simulink model "Manipulator_AdaptiveInverseDynamics"  (R2022b)
settings: Solver=FixedStepAuto  StartTime=0.0  StopTime=t_final  FixedStep=dt  RelTol=1e-3
values from neighbouring files (symbols this model uses):
  dt = 1.00e-03    (= 0.001)    [Initialization.m]
  Kd = 50*eye(3,3)    [AdaptiveInverseDynamicsInit.m]
  Kp = 20*eye(3,3)    [AdaptiveInverseDynamicsInit.m]
  P = lyap(A', Q)    [AdaptiveInverseDynamicsInit.m]
  theta_params_init = [p1;p2;p3;p4;p5;p6]    [AdaptiveInverseDynamicsInit.m]
libraries: simulink x3
settings Model: Creator=lukasz  LastModifiedBy=lukasz

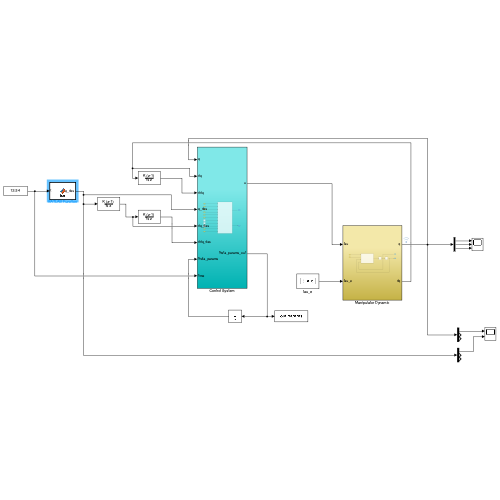
[thumbnail: Simulink's stored preview of the top-level diagram]
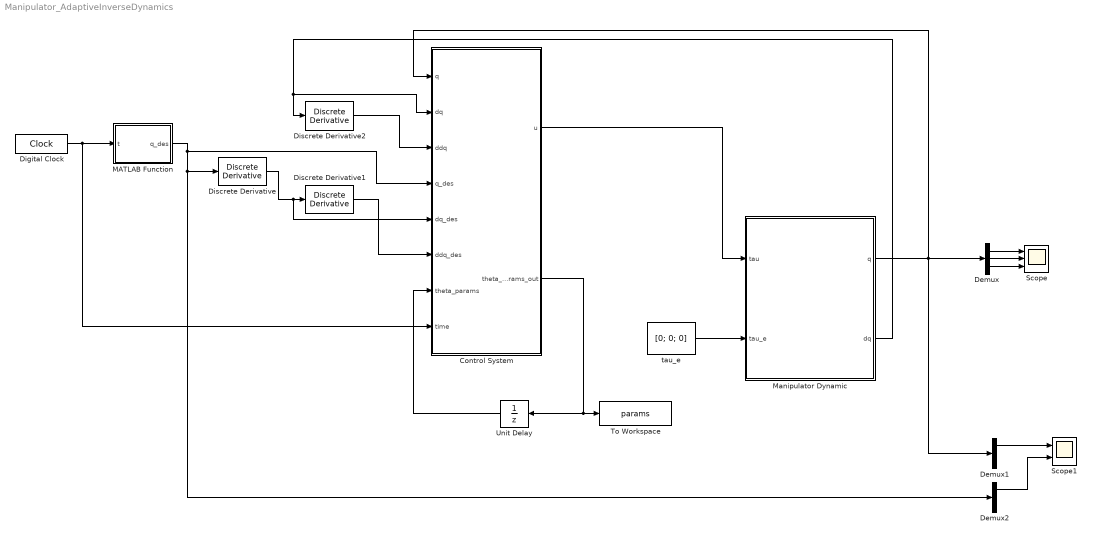
== system Manipulator_AdaptiveInverseDynamics ==
  Control System : Subsystem
  Demux : Demux  Outputs=3
  Demux1 : Demux  Outputs=3
  Demux2 : Demux  Outputs=3
  Digital Clock : DigitalClock  SampleTime=dt
  Discrete Derivative : simulink/Discrete/Discrete Derivative  gainval=1.0  ICPrevScaledInput=0  OutMin=[]  OutMax=[]  OutDataType=fixdt(1, 16)  OutScaling=2^-10  DoSatur=off
  Discrete Derivative1 : simulink/Discrete/Discrete Derivative  gainval=1  ICPrevScaledInput=0  OutMin=[]  OutMax=[]  OutDataType=fixdt(1, 16)  OutScaling=2^-10  DoSatur=off
  Discrete Derivative2 : simulink/Discrete/Discrete Derivative  gainval=1.0  ICPrevScaledInput=0  OutMin=[]  OutMax=[]  OutDataType=fixdt(1, 16)  OutScaling=2^-10  DoSatur=off
  MATLAB Function : MATLAB Function  TreatAsAtomicUnit=on
  Manipulator Dynamic : Subsystem
  Scope : Scope  NumInputPorts=3
  Scope1 : Scope  NumInputPorts=2
  To Workspace : ToWorkspace  VariableName=params  SaveFormat=Timeseries  SampleTime=-1
  Unit Delay : UnitDelay  InitialCondition=theta_params_init  SampleTime=-1  HasFrameUpgradeWarning=on
  tau_e : Constant  Value=[0; 0; 0]
  wires:
  MATLAB Function/1(q_des) -> Demux2/1, Discrete Derivative/1, Control System/4(q_des)
  Demux/3 -> Scope/3
  tau_e/1 -> Manipulator Dynamic/2(tau_e)
  Demux/1 -> Scope/1
  Discrete Derivative/1 -> Control System/5(dq_des), Discrete Derivative1/1
  Digital Clock/1 -> Control System/8(time), MATLAB Function/1(t)
  Discrete Derivative1/1 -> Control System/6(ddq_des)
  Demux/2 -> Scope/2
  Manipulator Dynamic/1(q) -> Control System/1(q), Demux/1, Demux1/1
  Demux1/1 -> Scope1/1
  Manipulator Dynamic/2(dq) -> Discrete Derivative2/1, Control System/2(dq)
  Demux2/1 -> Scope1/2
  Control System/1(u) -> Manipulator Dynamic/1(tau)
  Discrete Derivative2/1 -> Control System/3(ddq)
  Control System/2(theta_params_out) -> Unit Delay/1, To Workspace/1
  Unit Delay/1 -> Control System/7(theta_params)

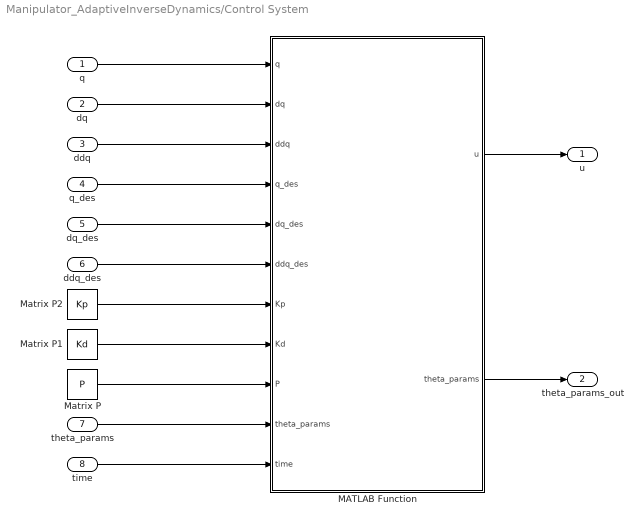
== system Manipulator_AdaptiveInverseDynamics/Control System ==
  q : Inport
  dq : Inport  Port=2
  ddq : Inport  Port=3
  q_des : Inport  Port=4
  dq_des : Inport  Port=5
  ddq_des : Inport  Port=6
  theta_params : Inport  Port=7
  time : Inport  Port=8
  MATLAB Function : MATLAB Function  TreatAsAtomicUnit=on
  Matrix P : Constant  Value=P
  Matrix P1 : Constant  Value=Kd
  Matrix P2 : Constant  Value=Kp
  u : Outport
  theta_params_out : Outport  Port=2
  wires:
  q_des/1 -> MATLAB Function/4(q_des)
  dq/1 -> MATLAB Function/2(dq)
  MATLAB Function/1(u) -> u/1
  q/1 -> MATLAB Function/1(q)
  dq_des/1 -> MATLAB Function/5(dq_des)
  ddq_des/1 -> MATLAB Function/6(ddq_des)
  time/1 -> MATLAB Function/11(time)
  ddq/1 -> MATLAB Function/3(ddq)
  MATLAB Function/2(theta_params) -> theta_params_out/1
  Matrix P2/1 -> MATLAB Function/7(Kp)
  Matrix P1/1 -> MATLAB Function/8(Kd)
  theta_params/1 -> MATLAB Function/10("theta_params ")
  Matrix P/1 -> MATLAB Function/9(P)

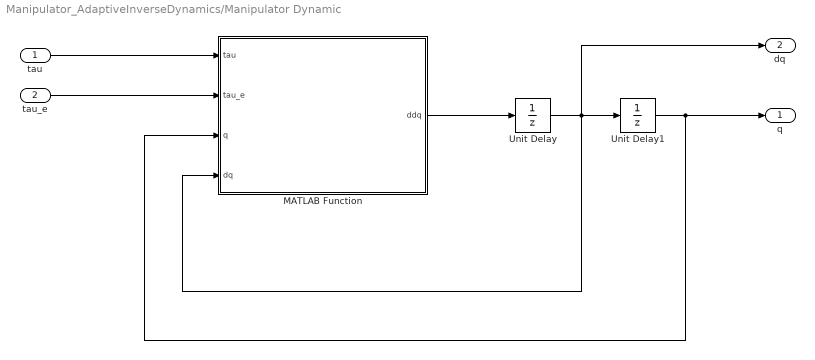
== system Manipulator_AdaptiveInverseDynamics/Manipulator Dynamic ==
  tau : Inport
  tau_e : Inport  Port=2
  MATLAB Function : MATLAB Function  TreatAsAtomicUnit=on
  Unit Delay : UnitDelay  InitialCondition=theta_params_init  SampleTime=-1  HasFrameUpgradeWarning=on
  Unit Delay1 : UnitDelay  InitialCondition=theta_params_init  SampleTime=-1  HasFrameUpgradeWarning=on
  q : Outport
  dq : Outport  Port=2
  wires:
  MATLAB Function/1(ddq) -> Unit Delay/1
  tau/1 -> MATLAB Function/1(tau)
  tau_e/1 -> MATLAB Function/2(tau_e)
  Unit Delay1/1 -> q/1, MATLAB Function/3(q)
  Unit Delay/1 -> Unit Delay1/1, dq/1, MATLAB Function/4(dq)

== matlab function Manipulator_AdaptiveInverseDynamics/Control System/MATLAB Function ==
  data: q input; u output; dq input; ddq input; q_des input; dq_des input; ddq_des input; Kp input; Kd input; P input; theta_params input; time input; theta_params output
function [u, theta_params]= AdaptiveInverseDynamics(q, dq, ddq, ...
                                     q_des, dq_des, ddq_des, ...
                                     Kp, Kd, ...
                                     P, theta_params, time)

%% reset first ddq_des
if (time < 0.003)
    qd_ddot = [0;0;0];
    qd_dot = [0;0;0];
end

%% Acceleration Control
ac = ddq_des - Kd*(dq - dq_des) - Kp*(q - q_des);

ddq1 = ac(1);
ddq2 = ac(2);
ddq3 = ac(3);

u = getYMatrix(q, dq, ac) * theta_params;

%% joint space variables
q1 = q(1);
q2 = q(2);
q3 = q(3);

dq1 = dq(1);
dq2 = dq(2);
dq3 = dq(3);

%% Parametric Form Matrix of Angular Quantities
Y_system = getYMatrix(q, dq, ddq);

%% Adaptive Parameter Estimation
% Gamma - learning rate of parameters
%Gamma = 0.1*eye(6,6);
Gamma = zeros(6,6);
Gamma(3,3) = 0.1;
Gamma(4,4) = 0.1;
% Estimated Inertia
H_hat = getHMatrix(q, theta_params);
B = [zeros(3,3); eye(3,3)];

% Errors
x = [q - q_des; dq - dq_des];

dTheta_params = -inv(Gamma)*Y_system.'*inv(H_hat)*(B.'*P*x);

%% Update theta parameters
dt = 0.001;
theta_params = theta_params + dTheta_params*dt;


function Y = getYMatrix(q, dq, ddq)
%% joint space variables
q1 = q(1);
q2 = q(2);
q3 = q(3);

dq1 = dq(1);
dq2 = dq(2);
dq3 = dq(3);

ddq1 = ddq(1);
ddq2 = ddq(2);
ddq3 = ddq(3);

Y11 = ddq1;
Y12 = sin(q2+q3)^2*ddq1 + sin(2*(q1+q2))*dq1*dq2 + sin(2*(q2+q3));
Y13 = cos(q2)^2-sin(2*q2)*dq1*dq2;
Y14 = 2*cos(q2)*sin(q2+q3)*ddq1 + 2*cos(2*q2+q3)*dq1*dq2 + 2*cos(q2)*cos(q2*q3);

Y22 = ddq2 + ddq3 - 0.5*sin(2*(q2+q3))*dq1^2;
Y23 = ddq2 + 0.5*sin(2*q2)*dq1^2;
Y24 = 2*sin(q3)*ddq2 + sin(q3)*ddq3 - cos(2*q2+q3)*dq1^2 + 2*cos(q3)*dq2*dq3 - cos(q3)*dq2*dq3^2;
Y25 = sin(q2+q3);
Y26 = cos(q2);

Y32 = ddq2 + ddq3 - 0.5*sin(2*(q2+q3))*dq1^2;
Y34 = sin(q3)*ddq2 - 0.5*cos(q2)*cos(q2+q3)*dq1^2 - cos(q3)*dq2^3;
Y35 = sin(q2+q3);

Y = [Y11, Y12, Y13, Y14,   0,   0;
       0, Y22, Y23, Y24, Y25, Y26;
       0, Y32,   0, Y34, Y35,   0];

function H = getHMatrix(q, theta_params)
% Parameters
q1 = q(1);
q2 = q(2);
q3 = q(3);

p1 = theta_params(1); % J
p2 = theta_params(2); % J1
p3 = theta_params(3); % J12
p4 = theta_params(4); % J13

h11 = p1 + p2*sin(q2+q3)^2 + p3*(cos(q2))^2 + 2*p4*cos(q2)*sin(q2+q3);
h22 = p2 + p3 + 2*p4*sin(q3);
h23 = p2 + p4*sin(q3);
h32 = h23;
h33 = p2;

H = [h11,   0,   0;
       0, h22, h23;
       0, h32, h33];

== matlab function Manipulator_AdaptiveInverseDynamics/Manipulator Dynamic/MATLAB Function ==
  data: tau input; tau_e input; q input; ddq output; dq input
function ddq = DynamicModel( tau, tau_e, q, dq)
%%%%%
% 3-DOF Puma-560 Dynamic Model Function
% H(q)* ddq + C(q) * dq + G = tau + tau_e
% q is 3*1 vector of joint variables (radian)
% H(q) is the inertia matrix
% C(q) is the matrix of Coriolis and centrifugal forces
% G(q) is  the vector of potential forces Parameters
% tau is control torque 
% tau_e is the external torque due to the interaction with the environment
%%%%%

%% Joint Space variables

q1 = q(1);
q2 = q(2);
q3 = q(3);

dq1 = dq(1);
dq2 = dq(2);
dq3 = dq(3);

%% general physical parameters

l1 = 0.6731;
l2 = 0.432;
l3 = 0.434;
lc2 = 0.216;
lc3 = 0.164;
m2 = 15.46;
m3 = 9.55;
J = 0.302;

%% Inertia Matrix Parameters

J1 = m3 * lc3^2;
J12 = (m2 * lc2^2) + (m3 * l2^2);
J13 = l2 * lc3 * m3;


h11 = J + J1 * (sin(q2 + q3))^2 + J12 * (cos(q2))^2 + 2 * J13 * cos(q2) * sin(q2+q3);
h22 = J1 + J12 + 2 * J13 * sin(q3);
h23 = J1 + J13 * sin(q3);
h32 = h23;
h33 = J1;

H = [h11, 0 ,0 ;
    0 , h22, h23;
    0 , h32, h33];

%% Coriolis Matrix Parameters

c12_1 = J1 * sin(2 * (q1 + q2)) - J12 * sin(2 * q2) + 2 * J13 * cos(2 * q2 +q3);
c13_1 = J1 * sin(2 * (q2 + q3)) + 2 * J13 * cos(q2) * cos(q2 + q3);
c11_2 = (1/2) * (-J1 * sin(2 * (q2 + q3)) + J12 * sin(2 * q2) - 2 * J13 * cos(2 * q2 + q3));
c22_2 = 2 * J13 * cos(q3);
c23_2 = J13 * cos(q3);
c22_3 = -J13 * cos(q3) * dq2;
c11_3 = (-1/2) * (J1 * sin(2 * (q2 + q3)) + J13 * cos(q2) * cos(q2 + q3));

C = [0, c12_1 * dq1, c13_1 * dq3;
    c11_2 * dq1, 0 , c22_2 * dq2 + c23_2 * dq3;
    c11_3 * dq1, c22_3 * dq2, 0];

%% Vector of Potential Forces Parameters

g = 9.81;

g21 = -g * (lc3 * m3 * sin(q2 + q3) + lc2 * m2 * cos(q2) + l2 * m3 * cos(q2));
g31 = -g * (lc3 * m3 * sin(q2 + q3));

G = [0;
    g21;
    g31];

%% Function output

ddq = inv(H)*(tau + tau_e - C * dq - G);
print(size(ddq))

== matlab function Manipulator_AdaptiveInverseDynamics/MATLAB Function ==
  data: t input; q_des output
function q_des = fcn(t)

q1 = (pi/4)*sin(t);
q2 = (pi/6) * cos(2*t + pi/4);
q3 = 0;

q_des = [q1; q2; q3];
